simulink model "Pacing"  (R2020a)
settings: Solver=FixedStepAuto  StartTime=0.0  StopTime=10.0  FixedStep=1e-3  RelTol=1e-3  EnableMultiTasking=on
undefined symbols (not defined in the file): D10, D11, D12, D2, D4, D5, D7, D8, D9, PTA0, PTA2, PTB23, PTB9, PTC3, PTC4, PTD0, PTD2, PTD3
libraries: frdmk64flib x34
settings Model: ExtModeTrigDuration=5  Creator=iceca  LastModifiedBy=iceca
settings OptimizationCC: EnhancedBackFolding=on  PassReuseOutputArgsAs=Individual arguments  ZeroExternalMemoryAtStartup=off  ZeroInternalMemoryAtStartup=off  MaxStackSize=64  OptimizeBlockOrder=speed  DifferentSizesBufferReuse=on  OptimizationCustomize=off  EfficientTunableParamExpr=on
settings DebuggingCC: ParameterTunabilityLossMsg=error
settings HardwareCC: ProdBitPerPointer=32  ProdBitPerSizeT=32  ProdBitPerPtrDiffT=32  ProdLargestAtomicInteger=Long  ProdLargestAtomicFloat=Double  ProdWordSize=32  ProdHWDeviceType=ARM Compatible->ARM Cortex
settings SFSimCC: MATLABDynamicMemAlloc=off
settings RTWCC: SystemTargetFile=ert.tlc  HardwareBoard=NXP FRDM-K64F  TemplateMakefile=ert_default_tmf  Toolchain=GNU Tools for ARM Embedded Processors
settings CodeAppCC: ForceParamTrailComments=on  IgnoreCustomStorageClasses=off  OperatorAnnotations=on  SimulinkDataObjDesc=on  SFDataObjDesc=on  InsertBlockDesc=on

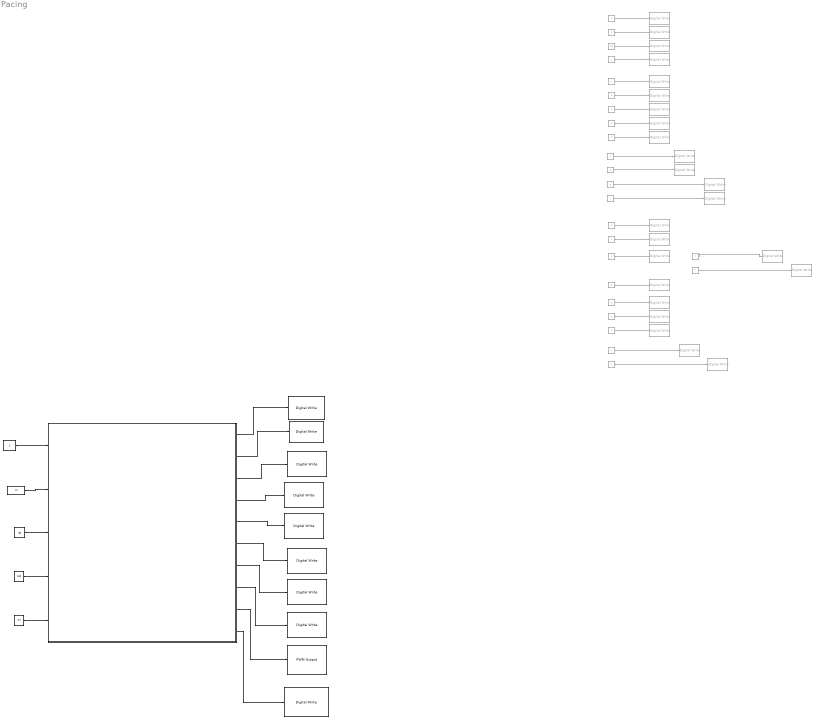
== system Pacing ==
  note: Charging C22
  note: AV Pacing
  note: Atrial Pacing
  note: Ventricular Pacing
  note: Discharging C21
  note: Atrial Pacing
  note: Ventricular Pacing
  Chart : Stateflow chart  TreatAsAtomicUnit=on
  Constant{,1,5..7,11..14,16..17,19..23} (16 alike) : Constant  Commented=on  Value=0
  Constant{3..4,8..10,15,18} (7 alike) : Constant  Commented=on
  Constant2 : Constant  Commented=on  Value=50
  Constant24 : Constant  Value=60
  Constant25 : Constant  Value=3.7
  Constant26 : Constant  Value=120
  Constant27 : Constant  Value=10
  Constant28 : Constant
  Digital Write{,9,14,20,23} (5 alike) : frdmk64flib/Digital Write  Commented=on  Whichpin=PTA0 (D8)
  Digital Write{1,8,11,21} (4 alike) : frdmk64flib/Digital Write  Commented=on  Whichpin=PTC4 (D9)
  Digital Write10 : frdmk64flib/Digital Write  Commented=on  Whichpin=PTD0 (D10)
  Digital Write12 : frdmk64flib/Digital Write  Commented=on  Whichpin=PTB23 (D4)
  Digital Write13 : frdmk64flib/Digital Write  Commented=on  Whichpin=PTC3 (D7)
  Digital Write15 : frdmk64flib/Digital Write  Commented=on  Whichpin=PTD2 (D11)
  Digital Write16 : frdmk64flib/Digital Write  Commented=on  Whichpin=PTD3 (D12)
  Digital Write17 : frdmk64flib/Digital Write  Commented=on  Whichpin=PTD2 (D11)
  Digital Write18 : frdmk64flib/Digital Write  Commented=on  Whichpin=PTD3 (D12)
  Digital Write19 : frdmk64flib/Digital Write  Commented=on  Whichpin=PTB9 (D2)
  Digital Write2 : frdmk64flib/Digital Write  Commented=on  Whichpin=PTA2 (D5)
  Digital Write22 : frdmk64flib/Digital Write  Commented=on  Whichpin=PTD2 (D11)
  Digital Write24 : frdmk64flib/Digital Write  Whichpin=PTB9 (D2)
  Digital Write25 : frdmk64flib/Digital Write  Whichpin=PTD0 (D10)
  Digital Write26 : frdmk64flib/Digital Write  Whichpin=PTA0 (D8)
  Digital Write27 : frdmk64flib/Digital Write  Whichpin=PTD2 (D11)
  Digital Write28 : frdmk64flib/Digital Write  Whichpin=PTB23 (D4)
  Digital Write29 : frdmk64flib/Digital Write  Whichpin=PTC3 (D7)
  Digital Write3 : frdmk64flib/Digital Write  Commented=on  Whichpin=PTB9 (D2)
  Digital Write30 : frdmk64flib/Digital Write  Whichpin=PTC4 (D9)
  Digital Write31 : frdmk64flib/Digital Write  Whichpin=PTD3 (D12)
  Digital Write32 : frdmk64flib/Digital Write  Whichpin=BLUE_LED
  Digital Write4 : frdmk64flib/Digital Write  Commented=on  Whichpin=PTD0 (D10)
  Digital Write5 : frdmk64flib/Digital Write  Commented=on  Whichpin=PTB23 (D4)
  Digital Write6 : frdmk64flib/Digital Write  Commented=on  Whichpin=PTC3 (D7)
  Digital Write7 : frdmk64flib/Digital Write  Commented=on  Whichpin=PTD3 (D12)
  PWM Output : frdmk64flib/PWM Output  Whichpin=PTA2 (D5)  InitialFrequency=2000  InitialDutyCycle=50
  wires:
  Constant/1 -> Digital Write/1
  Constant1/1 -> Digital Write1/1
  Constant2/1 -> Digital Write2/1
  Constant3/1 -> Digital Write3/1
  Constant10/1 -> Digital Write10/1
  Constant11/1 -> Digital Write11/1
  Constant12/1 -> Digital Write12/1
  Constant13/1 -> Digital Write13/1
  Constant14/1 -> Digital Write14/1
  Constant15/1 -> Digital Write15/1
  Constant16/1 -> Digital Write16/1
  Constant17/1 -> Digital Write17/1
  Constant18/1 -> Digital Write18/1
  Constant4/1 -> Digital Write4/1
  Constant5/1 -> Digital Write5/1
  Constant6/1 -> Digital Write6/1
  Constant7/1 -> Digital Write7/1
  Constant8/1 -> Digital Write8/1
  Constant9/1 -> Digital Write9/1
  Constant19/1 -> Digital Write19/1
  Constant20/1 -> Digital Write20/1
  Constant21/1 -> Digital Write21/1
  Constant22/1 -> Digital Write22/1
  Constant23/1 -> Digital Write23/1
  Chart/1(PACE_CHARGE_CTRL_D2) -> Digital Write24/1
  Chart/2(PACE_GND_CTRL_D10) -> Digital Write25/1
  Chart/3(ATR_PACE_CTRL_D8) -> Digital Write26/1
  Chart/4(ATR_GND_CTRL_D11) -> Digital Write27/1
  Chart/5(Z_ATR_CTRL_D4) -> Digital Write28/1
  Chart/6(Z_VENT_CTRL_D7) -> Digital Write29/1
  Chart/7(VENT_GND_CTRL_D12) -> Digital Write31/1
  Chart/8(VENT_PACE_CTRL_D9) -> Digital Write30/1
  Chart/9(PACING_REF_PWM_D5) -> PWM Output/1
  Constant28/1 -> Chart/1(Pacing_Mode)
  Constant25/1 -> Chart/5(Pulse_Amplitude)
  Constant26/1 -> Chart/4(Upper_Rate_Limit)
  Constant24/1 -> Chart/3(Lower_Rate_Limit)
  Constant27/1 -> Chart/2(Pulse_Width)
  Chart/10(LED_RED) -> Digital Write32/1

== stateflow chart Pacing/Chart ==
  state AV_Pacing_state_2
    entry:
    LED_RED = LOW;
    %PACING_REF_PWM_D5 = 75;
    %PACE_CHARGE_CTRL_D2 = LOW;
    %VENT_PACE_CTRL_D9 = HIGH;
    %VENT_GND_CTRL_D12 = LOW;
    %PACE_GND_CTRL_D10 = HIGH;
    %Z_VENT_CTRL_D7 = LOW;
    PACE_CHARGE_CTRL_D2 = LOW;
    PACE_GND_CTRL_D10 = HIGH;
    ATR_PACE_CTRL_D8 = LOW;
    ATR_GND_CTRL_D11 =LOW;
    Z_ATR_CTRL_D4 = LOW;
    Z_VENT_CTRL_D7 = LOW;
    VENT_GND_CTRL_D12 = LOW;
    if Pacing_Mode == 1
    VENT_PACE_CTRL_D9 =HIGH;
    else
    VENT_PACE_CTRL_D9 =LOW;
    ATR_PACE_CTRL_D8 =HIGH;
    end
  state Discharching_C21_and_Charging_C22
    entry:
    %charging C22
    LED_RED=HIGH;
    ATR_PACE_CTRL_D8   = LOW;
    VENT_PACE_CTRL_D9 = LOW;
    PACING_REF_PWM_D5 = Pulse_Amplitude*20;
    PACE_CHARGE_CTRL_D2 = HIGH;
    %discharching C21
    PACE_GND_CTRL_D10=HIGH;
    VENT_PACE_CTRL_D9=LOW;
    Z_ATR_CTRL_D4 = LOW;
    Z_VENT_CTRL_D7 = LOW;
    ATR_PACE_CTRL_D8 = LOW;
    if Pacing_Mode == 1
    VENT_GND_CTRL_D12 = HIGH;
    else
    ATR_GND_CTRL_D11 = HIGH;
    VENT_GND_CTRL_D12= LOW;
    end
    Rate = 60000/40 - Pulse_Width;
  (default) -> Discharching_C21_and_Charging_C22
  Discharching_C21_and_Charging_C22 -> AV_Pacing_state_2 : [after(300, msec)]
  AV_Pacing_state_2 -> Discharching_C21_and_Charging_C22 : [after(Pulse_Width, msec)]
  data: PACE_CHARGE_CTRL_D2 output; PACE_GND_CTRL_D10 output; ATR_PACE_CTRL_D8 output; ATR_GND_CTRL_D11 output; Z_ATR_CTRL_D4 output; Z_VENT_CTRL_D7 output; VENT_GND_CTRL_D12 output; VENT_PACE_CTRL_D9 output; Pacing_Mode input; PACING_REF_PWM_D5 output; Pulse_Width input double; avgRate local double; Lower_Rate_Limit input double; Upper_Rate_Limit input; Rate local double; Pulse_Amplitude input; HIGH local boolean =true; LOW local boolean =false; LED_RED output
